simulink model "zad4"  (R2022b)
settings: Solver=VariableStepAuto  StartTime=0.0  StopTime=100  RelTol=1e-3
values from neighbouring files (symbols this model uses):
  a0 = 0.000641026    [parameters.m]
  a1 = 0.0224359    [parameters.m]
  a2 = 0.260256    [parameters.m]
  Tp = 1    [parameters.m]
settings Model: Creator=Mat  LastModifiedBy=Mat

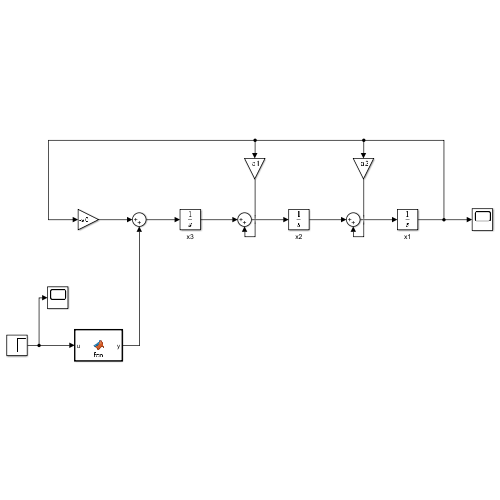
[thumbnail: Simulink's stored preview of the top-level diagram]
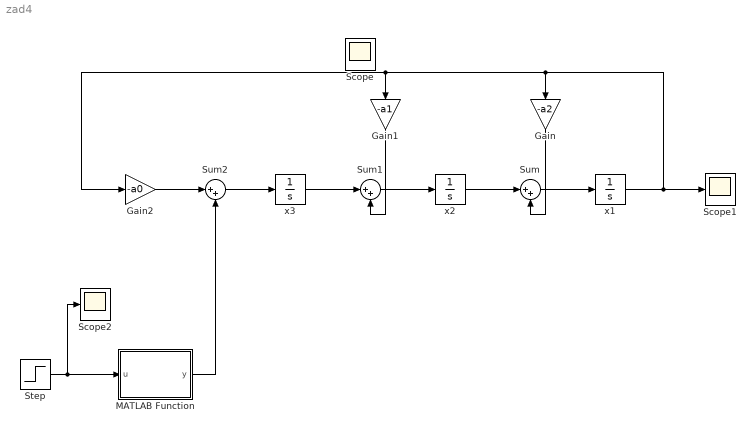
== system zad4 ==
  Gain : Gain  Gain=-a2
  Gain1 : Gain  Gain=-a1
  Gain2 : Gain  Gain=-a0
  MATLAB Function : MATLAB Function  TreatAsAtomicUnit=on
  Scope1 : Scope
  Scope2 : Scope
  Step : Step  Time=25  Before=-1  SampleTime=Tp
  Sum : Sum  Inputs=|++
  Sum1 : Sum  Inputs=|++
  Sum2 : Sum  Inputs=|++
  x1 : Integrator
  x2 : Integrator
  x3 : Integrator
  Scope : Scope
  wires:
  Sum2/1 -> x3/1
  Gain2/1 -> Sum2/1
  x1/1 -> Scope1/1, Gain1/1, Gain2/1, Gain/1
  x3/1 -> Sum1/1
  x2/1 -> Sum/1
  Sum/1 -> x1/1
  Sum1/1 -> x2/1
  Gain1/1 -> Sum1/2
  Gain/1 -> Sum/2
  Step/1 -> Scope2/1, MATLAB Function/1(u)
  MATLAB Function/1(y) -> Sum2/2

== matlab function zad4/MATLAB Function ==
  data: u input; y output
function y = fcn(u)
b0 = 0.000897436;
alfa1 = 1.3;
alfa2 = 1.1;
alfa3 = -1.15;
alfa4 = -0.9;
y = b0*(alfa1*u+alfa2*u^2+alfa3*u^3+alfa4*u^4);
end
